simulink model "boost_rom_mlp_v2_seed3"  (R2026a)
settings: Solver=ode1  StopTime=1.4  FixedStep=5e-07
PreLoadFcn:
  | mdlDir = fileparts(which('boost_rom_mlp_v2_seed3'));
  | repoRoot = fileparts(mdlDir);
  | load(fullfile(repoRoot, 'model_data', 'boost_rom_mlp_v2_seed3_data.mat'));
  | load(fullfile(repoRoot, 'model_data', 'comparison_duty_profile.mat'));
  | 
  | W = load(fullfile(repoRoot, 'model_data', 'mlp_v2_seed3_dlnetwork.mat'));
  | net_mlp = W.net_mlp;
values from neighbouring files (symbols this model uses):
  node_state_ic = [Vout_init; iL_init]    [setup_comparison_profile.m]
undefined symbols (not defined in the file or in its folder): lut_delta_iL, lut_duty, node_u_mean, node_u_std, node_x_mean, node_x_std
libraries: dlconvfclib x3, dlactivationlib x2
settings Model: SimulationMode=accelerator  Creator=arkadiyturevskiy  LastModifiedBy=arkadiyturevskiy

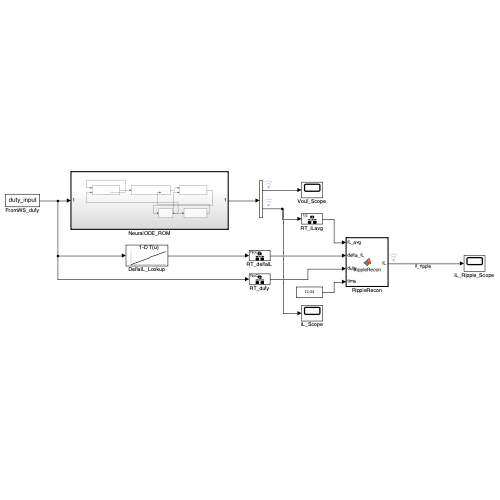
[thumbnail: Simulink's stored preview of the top-level diagram]
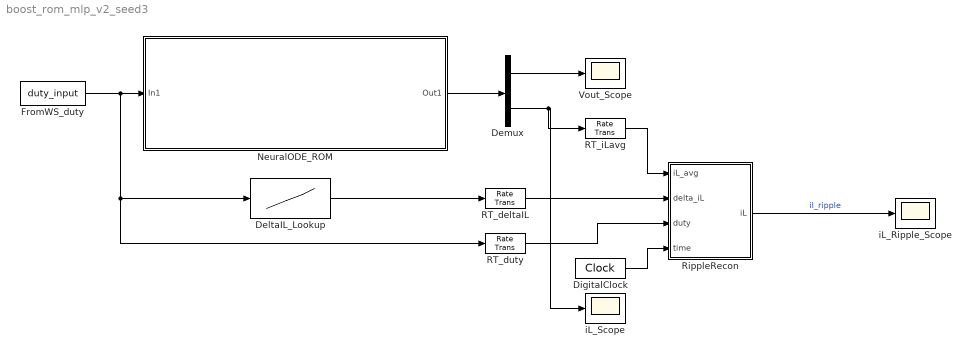
== system boost_rom_mlp_v2_seed3 ==
  DeltaIL_Lookup : Lookup_n-D  NumberOfTableDimensions=1  BreakpointsForDimension1=lut_duty  Table=lut_delta_iL  ExtrapMethod=Clip  InternalRulePriority=Speed  RndMeth=Simplest
  Demux : Demux  Outputs=2
  DigitalClock : DigitalClock  SampleTime=5e-07
  FromWS_duty : FromWorkspace  VariableName=duty_input  OutputAfterFinalValue=Holding final value
  NeuralODE_ROM : Subsystem  TreatAsAtomicUnit=on  SystemSampleTime=5e-06
  RT_deltaIL : RateTransition  OutPortSampleTime=5e-07
  RT_duty : RateTransition  OutPortSampleTime=5e-07
  RT_iLavg : RateTransition  OutPortSampleTime=5e-07
  RippleRecon : MATLAB Function  TreatAsAtomicUnit=on
  Vout_Scope : Scope
  iL_Ripple_Scope : Scope
  iL_Scope : Scope
  wires:
  DigitalClock/1 -> RippleRecon/4(time)
  RT_deltaIL/1 -> RippleRecon/2(delta_iL)
  Demux/1 -> Vout_Scope/1
  DeltaIL_Lookup/1 -> RT_deltaIL/1
  RippleRecon/1(iL) -> iL_Ripple_Scope/1  "il_ripple"
  Demux/2 -> RT_iLavg/1, iL_Scope/1
  RT_duty/1 -> RippleRecon/3(duty)
  NeuralODE_ROM/1(Out1) -> Demux/1
  RT_iLavg/1 -> RippleRecon/1(iL_avg)
  FromWS_duty/1 -> RT_duty/1, DeltaIL_Lookup/1, NeuralODE_ROM/1(In1)

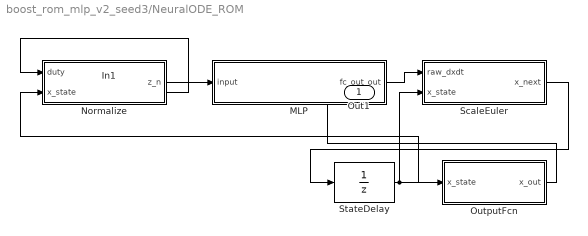
== system boost_rom_mlp_v2_seed3/NeuralODE_ROM ==
  In1 : Inport
  MLP : Subsystem
  Normalize : MATLAB Function  TreatAsAtomicUnit=on
  OutputFcn : MATLAB Function  TreatAsAtomicUnit=on
  ScaleEuler : MATLAB Function  TreatAsAtomicUnit=on
  StateDelay : UnitDelay  InitialCondition=node_state_ic  SampleTime=5e-06
  Out1 : Outport
  wires:
  In1/1 -> Normalize/1(duty)
  StateDelay/1 -> Normalize/2(x_state), ScaleEuler/2(x_state), OutputFcn/1(x_state)
  Normalize/1(z_n) -> MLP/1(input)
  MLP/1(fc_out_out) -> ScaleEuler/1(raw_dxdt)
  ScaleEuler/1(x_next) -> StateDelay/1
  OutputFcn/1(x_out) -> Out1/1

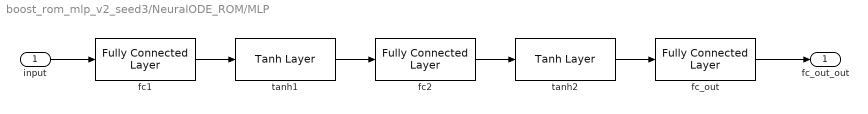
== system boost_rom_mlp_v2_seed3/NeuralODE_ROM/MLP ==
  input : Inport  PortDimensions=[3]  SampleTime=5e-06
  fc1 : dlconvfclib/Fully Connected Layer  Layer=net_mlp.Layers(2)  OutMin=[]  OutMax=[]  WeightsDataTypeStr=Inherit: Inherit via back propagation  WeightsMin=[]  WeightsMax=[]  BiasDataTypeStr=Inherit: Inherit via back propagation  BiasMin=[]  BiasMax=[]  AccumMin=[]  AccumMax=[]  InternalRndMeth=Floor  InternalSaturateOnIntegerOverflow=off  SampleTime=5e-06
      settings: DataFormat=C
  fc2 : dlconvfclib/Fully Connected Layer  Layer=net_mlp.Layers(4)  OutMin=[]  OutMax=[]  WeightsDataTypeStr=Inherit: Inherit via back propagation  WeightsMin=[]  WeightsMax=[]  BiasDataTypeStr=Inherit: Inherit via back propagation  BiasMin=[]  BiasMax=[]  AccumMin=[]  AccumMax=[]  InternalRndMeth=Floor  InternalSaturateOnIntegerOverflow=off  SampleTime=5e-06
      settings: DataFormat=C
  fc_out : dlconvfclib/Fully Connected Layer  Layer=net_mlp.Layers(6)  OutMin=[]  OutMax=[]  WeightsDataTypeStr=Inherit: Inherit via back propagation  WeightsMin=[]  WeightsMax=[]  BiasDataTypeStr=Inherit: Inherit via back propagation  BiasMin=[]  BiasMax=[]  AccumMin=[]  AccumMax=[]  InternalRndMeth=Floor  InternalSaturateOnIntegerOverflow=off  SampleTime=5e-06
      settings: DataFormat=C
  tanh1 : dlactivationlib/Tanh Layer  ApproximationMethod=None  OutMin=[]  OutMax=[]  SampleTime=5e-06
  tanh2 : dlactivationlib/Tanh Layer  ApproximationMethod=None  OutMin=[]  OutMax=[]  SampleTime=5e-06
  fc_out_out : Outport
  wires:
  fc2/1 -> tanh2/1
  input/1 -> fc1/1
  tanh2/1 -> fc_out/1
  fc_out/1 -> fc_out_out/1
  fc1/1 -> tanh1/1
  tanh1/1 -> fc2/1

== matlab function boost_rom_mlp_v2_seed3/NeuralODE_ROM/ScaleEuler ==
  data: raw_dxdt input; x_next output; x_state input; node_dxdt_scale parameter
function x_next = ScaleEuler(raw_dxdt, x_state, node_dxdt_scale)
%#codegen
Ts = 5.0000000000e-06;
dxdt = double(raw_dxdt) .* node_dxdt_scale;
x_next = x_state + Ts * dxdt;

== matlab function boost_rom_mlp_v2_seed3/NeuralODE_ROM/Normalize ==
  data: duty input; z_n output; x_state input; node_x_mean parameter; node_x_std parameter; node_u_mean parameter; node_u_std parameter
function z_n = Normalize(duty, x_state, node_x_mean, node_x_std, node_u_mean, node_u_std)
%#codegen
x_n = (x_state - node_x_mean) ./ node_x_std;
u_n = (duty - node_u_mean) / node_u_std;
z_n = single([x_n; u_n]);

== matlab function boost_rom_mlp_v2_seed3/NeuralODE_ROM/OutputFcn ==
  data: x_state input; x_out output
function x_out = OutputFcn(x_state)
%#codegen
x_out = x_state;

== matlab function boost_rom_mlp_v2_seed3/RippleRecon ==
  data: iL_avg input; iL output; delta_iL input; duty input; time input
function iL = RippleRecon(iL_avg, delta_iL, duty, time)
%#codegen
Tsw = 5.0000000000e-06;
phase = mod(time, Tsw) / Tsw;
duty_c = max(0.01, min(0.99, duty));
if phase < duty_c
    iL = iL_avg - delta_iL/2 + delta_iL * (phase / duty_c);
else
    iL = iL_avg + delta_iL/2 - delta_iL * ((phase - duty_c) / (1 - duty_c + eps));
end
